simulink model "Linear_ADMIRE_sim"  (Simulink 8.4)
settings: Solver=ode4  StartTime=0.0  StopTime=10  FixedStep=dt  RelTol=1e-3
InitFcn:
  | INIT_LINEAR
values from neighbouring files (symbols this model uses):
  a1 = (180*d2r)/(80^3)    (= 6.13592315154e-06)    [INIT_LINEAR.m]    (also in INIT_NDI.m)
  a2 = (24*d2r)/(80^3)    (= 8.18123086872e-07)    [INIT_LINEAR.m]    (also in INIT_NDI.m)
  a3 = (5*d2r)/(200)    (= 0.000436332312999)    [INIT_LINEAR.m]    (also in INIT_NDI.m)
  Abare = [-0.0369710265542 -0.00338320638614 0 0 0.00101076287488 0 0 0 0 1.00000000002 0 1.7763568394e-12 ... (784 elements, 28x28)]    [Trim_M0p22ALT20_LinDATA.mat]    (also in Trim_M0p3ALT2000_LinDATA.mat = [-0.0208061645292 -0.00191640084378 0 0 0.000610808752105 0 )
  Bbare = [-1.10043807057 0.00182125944543 -0.00701366565749 0.707306131876 1.12037014439 -0.330899025785 0 0 0 0 0 0 ... (448 elements, 28x16)]    [Trim_M0p22ALT20_LinDATA.mat]    (also in Trim_M0p3ALT2000_LinDATA.mat = [-1.42042676365 -0.000549876720984 -0.00633411409606 0.84954)
  CAmethod = 1    [ACA_init.m]    (also in INIT_LINEAR.m = 0; INIT_NDI.m = 0)
  Canard_max = interp1(M_vec,[25 25 25 15 15 15 15 15]*d2r,Mach,'next')    [INIT_LINEAR.m]    (also in INIT_NDI.m = [25 25 25 15 15 15 15 15]*d2r)
  Canard_min = interp1(M_vec,[-55 -55 -25 -15 -15 -15 -15 -15]*d2r,Mach,'next')    [INIT_LINEAR.m]    (also in INIT_NDI.m = [-55 -55 -25 -15 -15 -15 -15 -15]*d2r)
  CAobm = CAobm(:,1:12)    [INIT_LINEAR.m]
  Cbare = [1 0 0 0 0 0 0 0 0 0 0 0 ... (1652 elements, 59x28)]    [Trim_M0p22ALT20_LinDATA.mat]    (also in Trim_M0p3ALT2000_LinDATA.mat)
  CBobm = CCV*Bbare    [INIT_LINEAR.m]
  Dbare = [0 0 0 0 0 0 0 0 0 0 0 0 ... (944 elements, 59x16)]    [Trim_M0p22ALT20_LinDATA.mat]    (also in Trim_M0p3ALT2000_LinDATA.mat)
  dt = 0.01    [ACA_init.m]    (also in INIT_LINEAR.m; INIT_NDI.m)
  DTY_max = 0.002    [ACA_init.m]    (also in INIT_LINEAR.m; INIT_NDI.m)
  DTY_min = -0.002    [ACA_init.m]    (also in INIT_LINEAR.m; INIT_NDI.m)
  DTZ_max = 0.002    [ACA_init.m]    (also in INIT_LINEAR.m; INIT_NDI.m)
  DTZ_min = -0.002    [ACA_init.m]    (also in INIT_LINEAR.m; INIT_NDI.m)
  Elevon_max = interp1(M_vec,[30 30 25 25 25 25 25 25]*d2r,Mach,'next')    [INIT_LINEAR.m]    (also in INIT_NDI.m = [30 30 25 25 25 25 25 25]*d2r)
  Elevon_min = interp1(M_vec,[-30 -30 -30 -30 -30 -30 -30 -30]*d2r,Mach,'next')    [INIT_LINEAR.m]    (also in INIT_NDI.m = [-30 -30 -30 -30 -30 -30 -30 -30]*d2r)
  Fas_t = [0 1 1+dt 2. 2.+dt 8]    [INIT_LINEAR.m]
  Fas_v = [0 0 1 1 0 0]*40*0    [INIT_LINEAR.m]
  Fes_t = [0 1 1+dt 4 4+dt 7 7+dt 8]    [INIT_LINEAR.m]
  Fes_v = [0 0 1 1 -1 -1 0 0]*40    [INIT_LINEAR.m]
  Frp_t = [0 1 1+dt 6. 6.+dt 8]    [INIT_LINEAR.m]
  Frp_v = [0 0 1 1 0 0]*100*0    [INIT_LINEAR.m]
  G = [ 0 1 0 ... (first row only)    [ACA_init.m]    (also in INIT_LINEAR.m = [ 1 0 0; INIT_NDI.m)
  Kfb = -1.71    [INIT_LINEAR.m]
  Kfq = -3.4    [INIT_LINEAR.m]
  Kib = 5.14    [INIT_LINEAR.m]
  Kiq = 4    [INIT_LINEAR.m]
  Kp = 2.    (= 2)    [INIT_LINEAR.m]
  Kpb = 4.29    [INIT_LINEAR.m]
  Kpq = 3.4    [INIT_LINEAR.m]
  Kr = 14    [INIT_LINEAR.m]
  LEF_max = interp1(M_vec,[30 30 30 20 20 15 10 10]*d2r,Mach,'next')    [INIT_LINEAR.m]    (also in INIT_NDI.m = [30 30 30 20 20 15 10 10]*d2r)
  LEF_min = interp1(M_vec,[-10 -10 -10 -10 -10 -10 -10 -10]*d2r,Mach,'next')    [INIT_LINEAR.m]    (also in INIT_NDI.m = [-10 -10 -10 -10 -10 -10 -10 -10]*d2r)
  LG_max = 1    [ACA_init.m]    (also in INIT_LINEAR.m; INIT_NDI.m)
  LG_min = 0    [ACA_init.m]    (also in INIT_LINEAR.m; INIT_NDI.m)
  LPmethod = 3    [ACA_init.m]    (also in INIT_LINEAR.m = 0; INIT_NDI.m = 0; LPwrap.m = 0; LPwrap_1.m = 0)
  NumU = 16    [ACA_init.m]    (also in INIT_LINEAR.m; INIT_NDI.m; test.m; test_LPwrap.m)
  PD_max = 10    [ACA_init.m]    (also in INIT_LINEAR.m; INIT_NDI.m)
  PD_min = -10    [ACA_init.m]    (also in INIT_LINEAR.m; INIT_NDI.m)
  r2d = 180/pi    (= 57.2957795131)    [ACA_init.m]    (also in INIT_LINEAR.m; INIT_NDI.m)
  Rudder_max = interp1(M_vec,[30 30 25 20 15 15 15 10]*d2r,Mach,'next')    [INIT_LINEAR.m]    (also in INIT_NDI.m = [30 30 25 20 15 15 15 10]*d2r)
  Rudder_min = interp1(M_vec,[-30 -30 -25 -20 -15 -15 -15 -10]*d2r,Mach,'next')    [INIT_LINEAR.m]    (also in INIT_NDI.m = [-30 -30 -25 -20 -15 -15 -15 -10]*d2r)
  TSS_max = 1    [ACA_init.m]    (also in INIT_LINEAR.m; INIT_NDI.m)
  TSS_min = 0    [ACA_init.m]    (also in INIT_LINEAR.m; INIT_NDI.m)
  TSS_t = [0 1 1+dt 6. 6.+dt 8]    [INIT_LINEAR.m]
  TSS_v = [0 0 .1 .1 0 0]*0+u0new(10)    [INIT_LINEAR.m]
  UACTIVE = [ ... (first row only)    [INIT_LINEAR.m]
  UD_max = 10    [ACA_init.m]    (also in INIT_LINEAR.m; INIT_NDI.m)
  UD_min = -10    [ACA_init.m]    (also in INIT_LINEAR.m; INIT_NDI.m)
  Umax = [Canard_max*[1 1] Elevon_max*[1 1 1 1] Rudder_max LEF_max     LG_max TSS_max DTY_max DTZ_max UD_max VD_max WD_max PD_max]'    [INIT_LINEAR.m]    (also in INIT_NDI.m = [25 25 30 30 30 30 30]'*d2r)
  Umin = [Canard_min*[1 1] Elevon_min*[1 1 1 1] Rudder_min LEF_min     LG_min TSS_min DTY_min DTZ_min UD_min VD_min WD_min PD_min]'    [INIT_LINEAR.m]    (also in INIT_NDI.m = [-55 -55 -30 -30 -30 -30 -30]'*d2r)
  Unom = u0new    [INIT_LINEAR.m]
  Upref = [0 0 0 0 0 0 0 0 0 0 0 0 0 0 0 0]'    [ACA_init.m]    (also in INIT_LINEAR.m; INIT_NDI.m)
  UsePref = 0    [INIT_LINEAR.m]
  VD_max = 10    [ACA_init.m]    (also in INIT_LINEAR.m; INIT_NDI.m)
  VD_min = -10    [ACA_init.m]    (also in INIT_LINEAR.m; INIT_NDI.m)
  WD_max = 10    [ACA_init.m]    (also in INIT_LINEAR.m; INIT_NDI.m)
  WD_min = -10    [ACA_init.m]    (also in INIT_LINEAR.m; INIT_NDI.m)
  Wp = W'*W    [ACA_init.m]    (also in INIT_LINEAR.m; INIT_NDI.m; test.m; test_LPwrap.m)
  y0bare = [74.8477877145 0.159877852888 0 0 0 0 0 0.159877852888 0 0 0 -20 ... (73 elements, 73x1)]    [Trim_M0p22ALT20_LinDATA.mat]    (also in Trim_M0p3ALT2000_LinDATA.mat = [99.7587452043 0.116024082006 0 0 0 0 0 0.116024082006 0 0 0)
undefined symbols (not defined in the file or in its folder): CGIwrap, DAwrap, LPwrap, VJAwrap
libraries: simulink x6
(part 1 of 2)
settings Model: Creator=kenbordignon  LastModifiedBy=bordignk
settings DebuggingCC: CheckSSInitialOutputMsg=off  SolverPrmCheckMsg=none  UnconnectedInputMsg=none  UnconnectedOutputMsg=none  UnconnectedLineMsg=none

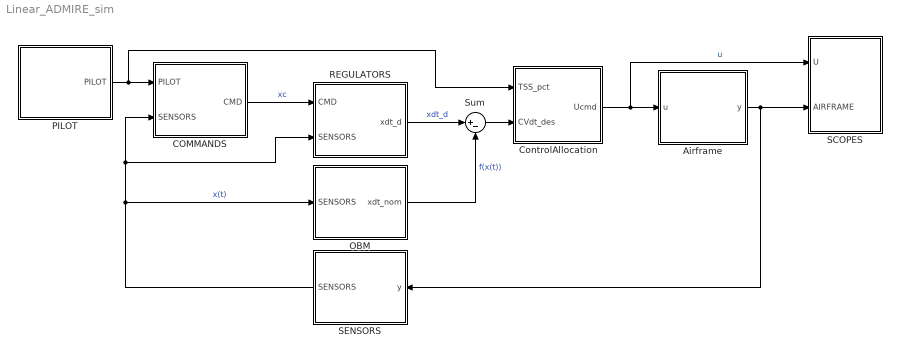
== system Linear_ADMIRE_sim ==
  Airframe : Subsystem
      mask Display: disp('AIRFRAME')
  COMMANDS : Subsystem
      mask Display: disp('COMMANDS')
  ControlAllocation : Subsystem
      mask Display: disp('CONTOL\nALLOCATION')
  OBM : Subsystem
      mask Display: disp('ON-BOARD\nMODEL')
  PILOT : Subsystem
      mask Display: disp('PILOT\nINCEPTORS')
  REGULATORS : Subsystem
      mask Display: disp('REGULATORS')
  SCOPES : Subsystem
      mask Display: disp('SCOPES\n&\nDISPLAYS')
  SENSORS : Subsystem
      mask Display: disp('SENSORS')
  Sum : Sum  Inputs=|+-
  wires:
  Airframe/1(y) -> SENSORS/1(y), SCOPES/2(AIRFRAME)
  SENSORS/1(SENSORS) -> OBM/1(SENSORS), REGULATORS/2(SENSORS), COMMANDS/2(SENSORS)  "x(t)"
  REGULATORS/1(xdt_d) -> Sum/1  "xdt_d"
  Sum/1 -> ControlAllocation/2(CVdt_des)
  COMMANDS/1(CMD) -> REGULATORS/1(CMD)  "xc"
  PILOT/1(PILOT) -> ControlAllocation/1(TSS_pct), COMMANDS/1(PILOT)
  ControlAllocation/1(Ucmd) -> Airframe/1(u), SCOPES/1(U)  "u"
  OBM/1(xdt_nom) -> Sum/2  "f(x(t))"

== system Linear_ADMIRE_sim/Airframe ==
  u : Inport
  A : Subsystem
      mask Display: disp('A')
  B : Subsystem
      mask Display: disp('B')
  C : Subsystem
      mask Display: disp('C')
  Constant4 : Constant  Value=Unom
  D : Subsystem
      mask Display: disp('D')
  Integrator : Integrator
  Sum : Sum  Inputs=|++
  Sum1 : Sum  Inputs=++|
  Sum2 : Sum  Inputs=|+-
  y : Outport
  wires:
  Integrator/1 -> C/1(In1), A/1(In1)  "x"
  B/1(Out1) -> Sum/1
  Sum/1 -> Integrator/1  "xdt"
  A/1(Out1) -> Sum/2
  Sum2/1 -> B/1(In1), D/1(In1)  "u"
  D/1(Out1) -> Sum1/1
  C/1(Out1) -> Sum1/2
  Sum1/1 -> y/1  "y"
  u/1 -> Sum2/1  "u"
  Constant4/1 -> Sum2/2

== system Linear_ADMIRE_sim/COMMANDS ==
  PILOT : Inport
  SENSORS : Inport  Port=2
  Bus Creator : BusCreator  Inputs=3
  PitchCmd : Subsystem
  RollCmd : Subsystem
  YawCmd : Subsystem
  CMD : Outport
  wires:
  PILOT/1 -> RollCmd/1(PILOT), YawCmd/1(PILOT), PitchCmd/1(PILOT)
  Bus Creator/1 -> CMD/1
  PitchCmd/1(Qc) -> Bus Creator/2
  RollCmd/1(Pc) -> Bus Creator/1
  YawCmd/1(Rc) -> Bus Creator/3
  SENSORS/1 -> YawCmd/2(SENSORS)

== system Linear_ADMIRE_sim/ControlAllocation ==
  TSS_pct : Inport
  CVdt_des : Inport  Port=2
  Bus Selector : BusSelector  OutputSignals=TSS_pct
  GetU : Subsystem
  PostProcess : Subsystem
  PreProcess : Subsystem
  Ucmd : Outport
  wires:
  PreProcess/1(PrePro) -> GetU/1(PrePro), PostProcess/2(PrePro)
  GetU/1(u) -> PostProcess/1(u)
  CVdt_des/1 -> PreProcess/1(CVdt_des)  "CVdt_des"
  PostProcess/1(Ucmd) -> Ucmd/1
  TSS_pct/1 -> Bus Selector/1
  Bus Selector/1 -> PostProcess/3(TSS_pct)  "<TSS_pct>"

== system Linear_ADMIRE_sim/OBM ==
  SENSORS : Inport
  Bus Selector : BusSelector  OutputSignals=VT_mps,ALPHA_rad,BETA_rad,P_rps,Q_rps,R_rps,PSI_rad,THETA_rad,PHI_rad,X_m,Y_m,Z_m  OutputAsBus=on
  Bus to Vector : BusToVector
  Gain1 : Gain  Gain=CAobm  Multiplication=Matrix(K*u)
  xdt_nom : Outport
  wires:
  SENSORS/1 -> Bus Selector/1
  Gain1/1 -> xdt_nom/1  "xdt_nom"
  Bus Selector/1 -> Bus to Vector/1  "x"
  Bus to Vector/1 -> Gain1/1

== system Linear_ADMIRE_sim/PILOT ==
  1-D Lookup Table : Lookup_n-D  NumberOfTableDimensions=1  BreakpointsForDimension1=Fas_t  Table=Fas_v  ExtrapMethod=Clip  UseLastTableValue=on  RndMeth=Simplest  InputSameDT=on
  1-D Lookup Table1 : Lookup_n-D  NumberOfTableDimensions=1  BreakpointsForDimension1=Fes_t  Table=Fes_v  ExtrapMethod=Clip  UseLastTableValue=on  RndMeth=Simplest  InputSameDT=on
  1-D Lookup Table2 : Lookup_n-D  NumberOfTableDimensions=1  BreakpointsForDimension1=Frp_t  Table=Frp_v  ExtrapMethod=Clip  UseLastTableValue=on  RndMeth=Simplest  InputSameDT=on
  1-D Lookup Table3 : Lookup_n-D  NumberOfTableDimensions=1  BreakpointsForDimension1=TSS_t  Table=TSS_v  ExtrapMethod=Clip  UseLastTableValue=on  RndMeth=Simplest  InputSameDT=on
  Bus Creator : BusCreator
  Clock : Clock
  Saturation : Saturate  UpperLimit=80  LowerLimit=-80
  Saturation1 : Saturate  UpperLimit=80  LowerLimit=-40
  Saturation2 : Saturate  UpperLimit=200  LowerLimit=-200
  Saturation3 : Saturate  UpperLimit=1  LowerLimit=0
  PILOT : Outport
  wires:
  Clock/1 -> 1-D Lookup Table/1, 1-D Lookup Table1/1, 1-D Lookup Table2/1, 1-D Lookup Table3/1
  1-D Lookup Table1/1 -> Saturation1/1
  1-D Lookup Table2/1 -> Saturation2/1
  1-D Lookup Table3/1 -> Saturation3/1
  Bus Creator/1 -> PILOT/1  "PILOT"
  Saturation/1 -> Bus Creator/1  "Fas_N"
  Saturation1/1 -> Bus Creator/2  "Fes_N"
  Saturation2/1 -> Bus Creator/3  "Frp_N"
  Saturation3/1 -> Bus Creator/4  "TSS_pct"
  1-D Lookup Table/1 -> Saturation/1

== system Linear_ADMIRE_sim/REGULATORS ==
  CMD : Inport
  SENSORS : Inport  Port=2
  Mux : Mux  Inputs=3
  PitchReg : Subsystem
  RollReg : Subsystem
  YawReg : Subsystem
  xdt_d : Outport
  wires:
  RollReg/1(Pdt_d) -> Mux/1
  PitchReg/1(Qdt_d) -> Mux/2
  YawReg/1(Rdt_d) -> Mux/3
  CMD/1 -> RollReg/1(CMD), PitchReg/1(CMD), YawReg/1(CMD)
  Mux/1 -> xdt_d/1  "xdt_d"
  SENSORS/1 -> RollReg/2(SENSORS), PitchReg/2(SENSORS), YawReg/2(SENSORS)

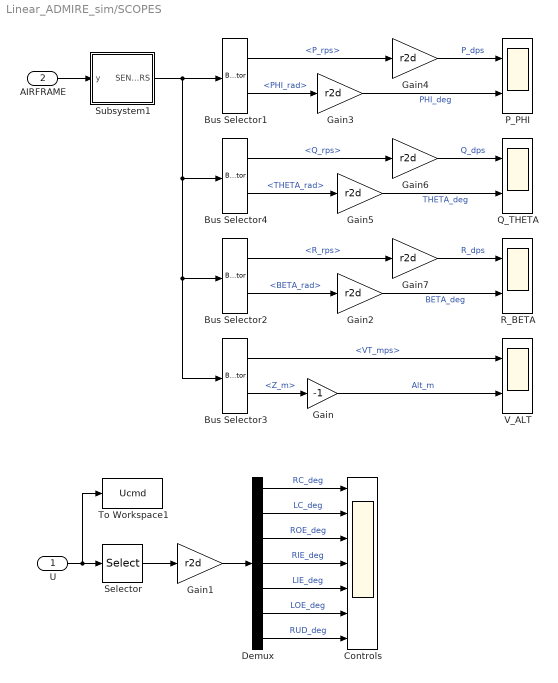
== system Linear_ADMIRE_sim/SCOPES ==
  U : Inport
  AIRFRAME : Inport  Port=2
  Bus Selector1 : BusSelector  OutputSignals=P_rps,PHI_rad
  Bus Selector2 : BusSelector  OutputSignals=R_rps,BETA_rad
  Bus Selector3 : BusSelector  OutputSignals=VT_mps,Z_m
  Bus Selector4 : BusSelector  OutputSignals=Q_rps,THETA_rad
  Controls : Scope  NumInputPorts=7
      settings: TimeRange=10  YMin=-10~-10~-5~-5~-5~-5~-5  YMax=5~5~5~5~5~5~5  SaveName=ScopeData2
  Demux : Demux  Outputs=7
  Gain : Gain  Gain=-1
  Gain{1..7} (7 alike) : Gain  Gain=r2d
  P_PHI : Scope  NumInputPorts=2
      settings: TimeRange=10  YMin=0~0  YMax=20~30
  Q_THETA : Scope  NumInputPorts=2
      settings: TimeRange=10  YMin=-4~8  YMax=4~18  SaveName=ScopeData4
  R_BETA : Scope  NumInputPorts=2
      settings: TimeRange=10  YMin=-10~-1  YMax=10~3
  Selector : Selector  InputPortWidth=16  Indices=[1:7]
  Subsystem1 : Subsystem
  To Workspace1 : ToWorkspace  VariableName=Ucmd  SampleTime=-1
  V_ALT : Scope  NumInputPorts=2
      settings: TimeRange=10  YMin=70~10  YMax=76~50  SaveName=ScopeData3
  wires:
  Subsystem1/1(SENSORS) -> Bus Selector3/1, Bus Selector2/1, Bus Selector4/1, Bus Selector1/1
  Bus Selector1/1 -> Gain4/1  "<P_rps>"
  AIRFRAME/1 -> Subsystem1/1(y)
  Bus Selector2/2 -> Gain2/1  "<BETA_rad>"
  Bus Selector1/2 -> Gain3/1  "<PHI_rad>"
  Bus Selector3/1 -> V_ALT/1  "<VT_mps>"
  Bus Selector3/2 -> Gain/1  "<Z_m>"
  Gain/1 -> V_ALT/2  "Alt_m"
  Selector/1 -> Gain1/1
  U/1 -> Selector/1, To Workspace1/1
  Demux/2 -> Controls/2  "LC_deg"
  Demux/3 -> Controls/3  "ROE_deg"
  Demux/4 -> Controls/4  "RIE_deg"
  Demux/5 -> Controls/5  "LIE_deg"
  Demux/6 -> Controls/6  "LOE_deg"
  Demux/7 -> Controls/7  "RUD_deg"
  Gain1/1 -> Demux/1
  Gain2/1 -> R_BETA/2  "BETA_deg"
  Gain3/1 -> P_PHI/2  "PHI_deg"
  Gain4/1 -> P_PHI/1  "P_dps"
  Bus Selector4/1 -> Gain6/1  "<Q_rps>"
  Bus Selector4/2 -> Gain5/1  "<THETA_rad>"
  Gain5/1 -> Q_THETA/2  "THETA_deg"
  Gain6/1 -> Q_THETA/1  "Q_dps"
  Gain7/1 -> R_BETA/1  "R_dps"
  Bus Selector2/1 -> Gain7/1  "<R_rps>"
  Demux/1 -> Controls/1  "RC_deg"

== system Linear_ADMIRE_sim/SENSORS ==
  note: Select 1:12 for actual values
      |
      | Select 32:43 for sensor approximations
  y : Inport
  Bus Creator : BusCreator  Inputs=12
  Demux : Demux  Outputs=12
  Selector : Selector  InputPortWidth=59  Indices=SensorIDX
  Unit Delay : UnitDelay  SampleTime=dt
  SENSORS : Outport
  wires:
  Demux/1 -> Bus Creator/1  "VT_mps"
  Demux/2 -> Bus Creator/2  "ALPHA_rad"
  Demux/3 -> Bus Creator/3  "BETA_rad"
  Demux/4 -> Bus Creator/4  "P_rps"
  Demux/5 -> Bus Creator/5  "Q_rps"
  Demux/6 -> Bus Creator/6  "R_rps"
  Demux/7 -> Bus Creator/7  "PSI_rad"
  Demux/8 -> Bus Creator/8  "THETA_rad"
  Demux/9 -> Bus Creator/9  "PHI_rad"
  Demux/10 -> Bus Creator/10  "X_m"
  Demux/11 -> Bus Creator/11  "Y_m"
  Demux/12 -> Bus Creator/12  "Z_m"
  y/1 -> Unit Delay/1
  Bus Creator/1 -> SENSORS/1
  Selector/1 -> Demux/1
  Unit Delay/1 -> Selector/1

== system Linear_ADMIRE_sim/Airframe/A ==
  In1 : Inport
  Gain1 : Gain  Gain=Abare  Multiplication=Matrix(K*u)
  Out1 : Outport
  wires:
  In1/1 -> Gain1/1
  Gain1/1 -> Out1/1

== system Linear_ADMIRE_sim/Airframe/B ==
  In1 : Inport
  Gain : Gain  Gain=Bbare  Multiplication=Matrix(K*u)
  Out1 : Outport
  wires:
  In1/1 -> Gain/1
  Gain/1 -> Out1/1

== system Linear_ADMIRE_sim/Airframe/C ==
  In1 : Inport
  Gain3 : Gain  Gain=Cbare  Multiplication=Matrix(K*u)
  Out1 : Outport
  wires:
  In1/1 -> Gain3/1
  Gain3/1 -> Out1/1

== system Linear_ADMIRE_sim/Airframe/D ==
  In1 : Inport
  Gain2 : Gain  Gain=Dbare  Multiplication=Matrix(K*u)
  Out1 : Outport
  wires:
  In1/1 -> Gain2/1
  Gain2/1 -> Out1/1

== system Linear_ADMIRE_sim/COMMANDS/PitchCmd ==
  PILOT : Inport
  Bus Selector1 : BusSelector  OutputSignals=Fes_N
  QCMD_Gradient : Lookup_n-D  NumberOfTableDimensions=1  BreakpointsForDimension1=[-80:80]  Table=a2*([-80:80].^3)  ExtrapMethod=Clip  UseLastTableValue=on  RndMeth=Simplest  InputSameDT=on
  Qc : Outport
  wires:
  PILOT/1 -> Bus Selector1/1
  Bus Selector1/1 -> QCMD_Gradient/1  "<Fes_N>"
  QCMD_Gradient/1 -> Qc/1  "Qc_rps"

== system Linear_ADMIRE_sim/COMMANDS/RollCmd ==
  PILOT : Inport
  Bus Selector2 : BusSelector  OutputSignals=Fas_N
  Gain4 : Gain  Gain=r2d
  PCMD_Gradient : Lookup_n-D  NumberOfTableDimensions=1  BreakpointsForDimension1=[-80:80]  Table=a1*([-80:80].^3)  ExtrapMethod=Clip  UseLastTableValue=on  RndMeth=Simplest  InputSameDT=on
  PC_dps : Scope
      settings: TimeRange=10  YMin=-50  YMax=50  SaveName=ScopeData8
  Pc : Outport
  wires:
  PILOT/1 -> Bus Selector2/1
  Bus Selector2/1 -> PCMD_Gradient/1  "<Fas_N>"
  PCMD_Gradient/1 -> Pc/1, Gain4/1  "Pc_rps"
  Gain4/1 -> PC_dps/1

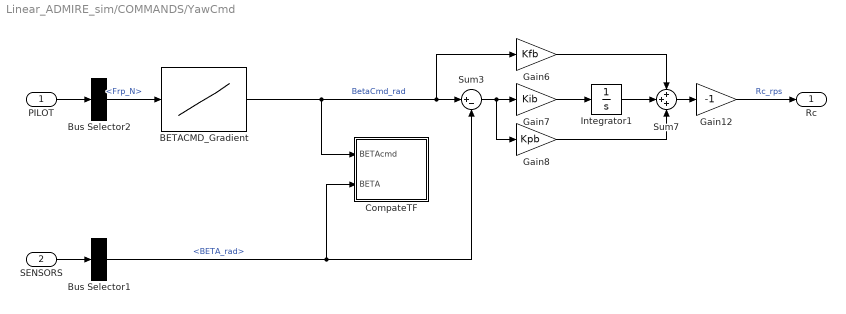
== system Linear_ADMIRE_sim/COMMANDS/YawCmd ==
  PILOT : Inport
  SENSORS : Inport  Port=2
  BETACMD_Gradient : Lookup_n-D  NumberOfTableDimensions=1  BreakpointsForDimension1=[-200 200]  Table=a3*([-200 200])  ExtrapMethod=Clip  UseLastTableValue=on  RndMeth=Simplest  InputSameDT=on
  Bus Selector1 : BusSelector  OutputSignals=BETA_rad
  Bus Selector2 : BusSelector  OutputSignals=Frp_N
  CompateTF : Subsystem
  Gain12 : Gain  Gain=-1
  Gain6 : Gain  Gain=Kfb
  Gain7 : Gain  Gain=Kib
  Gain8 : Gain  Gain=Kpb
  Integrator1 : Integrator
  Sum3 : Sum  Inputs=|+-
  Sum7 : Sum  Inputs=+++
  Rc : Outport
  wires:
  Sum7/1 -> Gain12/1
  Gain6/1 -> Sum7/1
  Gain7/1 -> Integrator1/1
  Sum3/1 -> Gain7/1, Gain8/1
  Gain8/1 -> Sum7/3
  Integrator1/1 -> Sum7/2
  Gain12/1 -> Rc/1  "Rc_rps"
  PILOT/1 -> Bus Selector2/1
  SENSORS/1 -> Bus Selector1/1
  Bus Selector1/1 -> Sum3/2, CompateTF/2(BETA)  "<BETA_rad>"
  Bus Selector2/1 -> BETACMD_Gradient/1  "<Frp_N>"
  BETACMD_Gradient/1 -> Sum3/1, Gain6/1, CompateTF/1(BETAcmd)  "BetaCmd_rad"

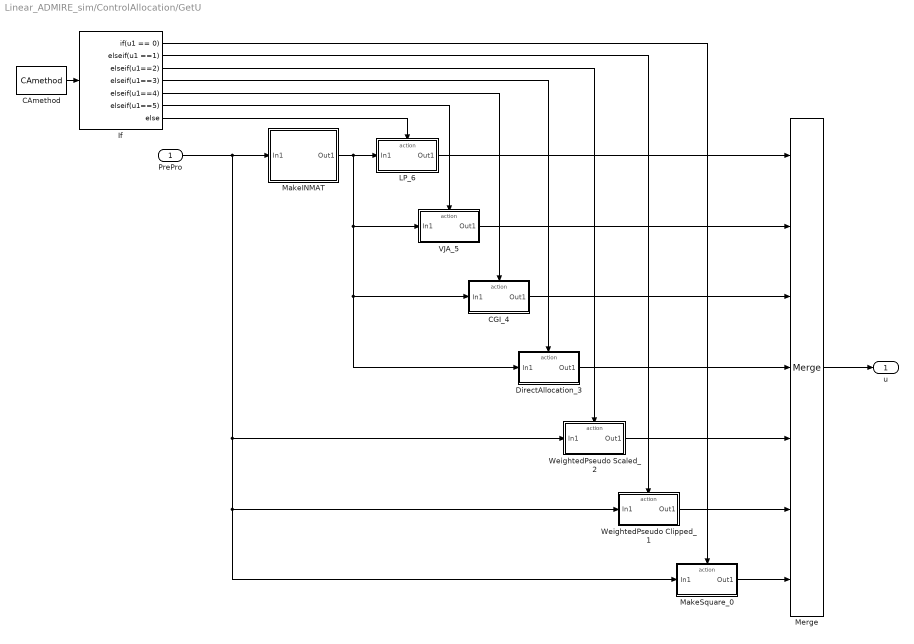
== system Linear_ADMIRE_sim/ControlAllocation/GetU ==
  PrePro : Inport
  CAmethod : Constant  Value=CAmethod  OutDataTypeStr=int8
  CGI_4 : Subsystem  TreatAsAtomicUnit=on
  DirectAllocation_3 : Subsystem  TreatAsAtomicUnit=on
  If : If  IfExpression=u1 == 0  ElseIfExpressions=u1 ==1, u1==2, u1==3, u1==4, u1==5
  LP_6 : Subsystem  TreatAsAtomicUnit=on
  MakeINMAT : Subsystem
  MakeSquare_0 : Subsystem  TreatAsAtomicUnit=on
  Merge : Merge  Inputs=7
  VJA_5 : Subsystem  TreatAsAtomicUnit=on
  WeightedPseudo Clipped_1 : Subsystem  TreatAsAtomicUnit=on
  WeightedPseudo Scaled_2 : Subsystem  TreatAsAtomicUnit=on
  u : Outport
  wires:
  CAmethod/1 -> If/1
  If/1 -> MakeSquare_0/Action
  If/2 -> WeightedPseudo Clipped_1/Action
  If/3 -> WeightedPseudo Scaled_2/Action
  If/4 -> DirectAllocation_3/Action
  VJA_5/1(Out1) -> Merge/2
  MakeSquare_0/1(Out1) -> Merge/7
  WeightedPseudo Clipped_1/1(Out1) -> Merge/6
  WeightedPseudo Scaled_2/1(Out1) -> Merge/5
  DirectAllocation_3/1(Out1) -> Merge/4
  If/5 -> CGI_4/Action
  CGI_4/1(Out1) -> Merge/3
  If/6 -> VJA_5/Action
  Merge/1 -> u/1
  If/7 -> LP_6/Action
  LP_6/1(Out1) -> Merge/1
  PrePro/1 -> MakeINMAT/1(In1), WeightedPseudo Scaled_2/1(In1), WeightedPseudo Clipped_1/1(In1), MakeSquare_0/1(In1)
  MakeINMAT/1(Out1) -> LP_6/1(In1), VJA_5/1(In1), DirectAllocation_3/1(In1), CGI_4/1(In1)

== system Linear_ADMIRE_sim/ControlAllocation/PostProcess ==
  u : Inport
  PrePro : Inport  Port=2
  TSS_pct : Inport  Port=3
  Bus Selector1 : BusSelector  OutputSignals=Unom
  DriveToPreferred : Subsystem
  LimitCommands : Subsystem
  Sum2 : Sum  Inputs=|++
  Sum3 : Sum  Inputs=|++
  Ucmd : Outport
  wires:
  Sum2/1 -> Sum3/1
  Sum3/1 -> LimitCommands/1(In1)
  u/1 -> DriveToPreferred/2(u), Sum2/1
  PrePro/1 -> DriveToPreferred/1(PrePro), Bus Selector1/1
  LimitCommands/1(Ucmd) -> Ucmd/1
  Bus Selector1/1 -> Sum2/2  "<Unom>"
  DriveToPreferred/1(Out2) -> Sum3/2
  TSS_pct/1 -> LimitCommands/2(TSS_pct)

== system Linear_ADMIRE_sim/ControlAllocation/PreProcess ==
  note: Data which usually comes from an
      | On-board Model and is assumed
      | constant for this simulation
  CVdt_des : Inport
  Bus Creator : BusCreator  Inputs=6
  Bus Creator1 : BusCreator
  Bus Selector1 : BusSelector  OutputSignals=CB,Unom,Umax,Umin
  Constant : Constant  Value=UACTIVE
  Constant1 : Constant  Value=CBobm
  Constant2 : Constant  Value=Umax
  Constant3 : Constant  Value=Umin
  Constant4 : Constant  Value=Unom
  PrePro : Outport
  wires:
  CVdt_des/1 -> Bus Creator/1
  Bus Creator/1 -> PrePro/1
  Constant/1 -> Bus Creator/6  "INDX"
  Constant1/1 -> Bus Creator1/1  "CB"
  Constant2/1 -> Bus Creator1/2  "Umax"
  Constant3/1 -> Bus Creator1/3  "Umin"
  Constant4/1 -> Bus Creator1/4  "Unom"
  Bus Creator1/1 -> Bus Selector1/1
  Bus Selector1/1 -> Bus Creator/2  "<CB>"
  Bus Selector1/2 -> Bus Creator/3  "<Unom>"
  Bus Selector1/3 -> Bus Creator/4  "<Umax>"
  Bus Selector1/4 -> Bus Creator/5  "<Umin>"

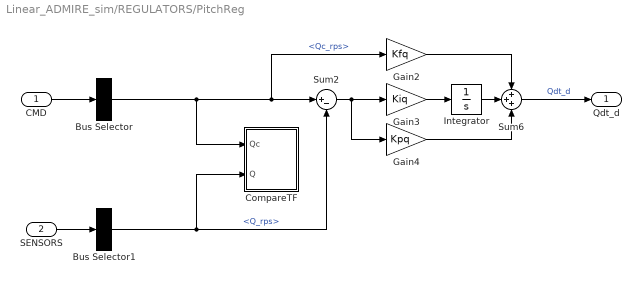
== system Linear_ADMIRE_sim/REGULATORS/PitchReg ==
  CMD : Inport
  SENSORS : Inport  Port=2
  Bus Selector : BusSelector  OutputSignals=Qc_rps
  Bus Selector1 : BusSelector  OutputSignals=Q_rps
  CompareTF : Subsystem
  Gain2 : Gain  Gain=Kfq
  Gain3 : Gain  Gain=Kiq
  Gain4 : Gain  Gain=Kpq
  Integrator : Integrator
  Sum2 : Sum  Inputs=|+-
  Sum6 : Sum  Inputs=+++
  Qdt_d : Outport
  wires:
  Sum2/1 -> Gain3/1, Gain4/1
  Gain3/1 -> Integrator/1
  Integrator/1 -> Sum6/2
  Gain4/1 -> Sum6/3
  Gain2/1 -> Sum6/1
  Bus Selector1/1 -> Sum2/2, CompareTF/2(Q)  "<Q_rps>"
  SENSORS/1 -> Bus Selector1/1
  Bus Selector/1 -> Sum2/1, Gain2/1, CompareTF/1(Qc)  "<Qc_rps>"
  Sum6/1 -> Qdt_d/1  "Qdt_d"
  CMD/1 -> Bus Selector/1

== system Linear_ADMIRE_sim/REGULATORS/RollReg ==
  CMD : Inport
  SENSORS : Inport  Port=2
  Bus Selector : BusSelector  OutputSignals=Pc_rps
  Bus Selector1 : BusSelector  OutputSignals=P_rps
  CompareTF : Subsystem
  Gain : Gain  Gain=Kp
  Sum8 : Sum  Inputs=|+-
  Pdt_d : Outport
  wires:
  Sum8/1 -> Gain/1
  Bus Selector1/1 -> Sum8/2, CompareTF/2(P)  "<P_rps>"
  SENSORS/1 -> Bus Selector1/1
  Gain/1 -> Pdt_d/1  "Pdt_d"
  CMD/1 -> Bus Selector/1
  Bus Selector/1 -> Sum8/1, CompareTF/1(Pc)  "<Pc_rps>"

== system Linear_ADMIRE_sim/REGULATORS/YawReg ==
  CMD : Inport
  SENSORS : Inport  Port=2
  Bus Selector : BusSelector  OutputSignals=Rc_rps
  Bus Selector1 : BusSelector  OutputSignals=R_rps
  CompareTF : Subsystem
  Gain5 : Gain  Gain=Kr
  Sum4 : Sum  Inputs=|+-
  Rdt_d : Outport
  wires:
  Sum4/1 -> Gain5/1
  Gain5/1 -> Rdt_d/1  "Rdt_d"
  CMD/1 -> Bus Selector/1
  SENSORS/1 -> Bus Selector1/1
  Bus Selector1/1 -> CompareTF/2(R), Sum4/2  "<R_rps>"
  Bus Selector/1 -> Sum4/1, CompareTF/1(Rc)  "<Rc_rps>"

== system Linear_ADMIRE_sim/SCOPES/Subsystem1 ==
  note: Select 1:12 for actual values
      |
      | Select 32:43 for sensor approximations
  note: Add in the trim conditions
  y : Inport
  Bus Creator : BusCreator  Inputs=12
  Constant : Constant  Value=y0bare(1:12)
  Demux : Demux  Outputs=12
  Selector : Selector  InputPortWidth=59  Indices=[1:12]
  Sum : Sum  Inputs=|++
  SENSORS : Outport
  wires:
  Demux/1 -> Bus Creator/1  "VT_mps"
  Demux/2 -> Bus Creator/2  "ALPHA_rad"
  Demux/3 -> Bus Creator/3  "BETA_rad"
  Demux/4 -> Bus Creator/4  "P_rps"
  Demux/5 -> Bus Creator/5  "Q_rps"
  Demux/6 -> Bus Creator/6  "R_rps"
  Demux/7 -> Bus Creator/7  "PSI_rad"
  Demux/8 -> Bus Creator/8  "THETA_rad"
  Demux/9 -> Bus Creator/9  "PHI_rad"
  Demux/10 -> Bus Creator/10  "X_m"
  Demux/11 -> Bus Creator/11  "Y_m"
  Demux/12 -> Bus Creator/12  "Z_m"
  y/1 -> Selector/1
  Bus Creator/1 -> SENSORS/1
  Sum/1 -> Demux/1
  Constant/1 -> Sum/2
  Selector/1 -> Sum/1

== system Linear_ADMIRE_sim/COMMANDS/YawCmd/CompateTF ==
  BETAcmd : Inport
  BETA : Inport  Port=2
  BetaTF_Beta : Scope
      settings: TimeRange=10  YMin=-1  YMax=3  SaveName=ScopeData6
  Gain2 : Gain  Gain=r2d
  Gain3 : Gain  Gain=r2d
  Mux1 : Mux  Inputs=2
  Scope2 : Scope
      settings: TimeRange=10  YMin=-6  YMax=1  SaveName=ScopeData7
  Sum2 : Sum  Inputs=|+-
  Transfer Fcn : TransferFcn  Numerator=[Kr*(Kfb+Kpb) Kr*Kib]  Denominator=[1 Kr Kr*Kpb Kr*Kib]
  Unit Delay : UnitDelay  SampleTime=dt
  wires:
  Mux1/1 -> Gain3/1
  Transfer Fcn/1 -> Unit Delay/1
  Sum2/1 -> Gain2/1
  Gain2/1 -> Scope2/1
  Gain3/1 -> BetaTF_Beta/1
  BETAcmd/1 -> Transfer Fcn/1
  BETA/1 -> Mux1/2, Sum2/2
  Unit Delay/1 -> Mux1/1, Sum2/1

== system Linear_ADMIRE_sim/ControlAllocation/GetU/CGI_4 ==
  In1 : Inport
  Action Port : ActionPort  ActionType=elseif
  MATLAB Fcn : MATLABFcn  MATLABFcn=CGIwrap(u)
  Out1 : Outport
  wires:
  MATLAB Fcn/1 -> Out1/1
  In1/1 -> MATLAB Fcn/1

== system Linear_ADMIRE_sim/ControlAllocation/GetU/DirectAllocation_3 ==
  In1 : Inport
  Action Port : ActionPort  ActionType=elseif
  MATLAB Fcn : MATLABFcn  MATLABFcn=DAwrap(u)
  Out1 : Outport
  wires:
  MATLAB Fcn/1 -> Out1/1
  In1/1 -> MATLAB Fcn/1

== system Linear_ADMIRE_sim/ControlAllocation/GetU/LP_6 ==
  In1 : Inport
  Action Port : ActionPort  ActionType=else
  MATLAB Fcn : MATLABFcn  MATLABFcn=LPwrap(u)
  Out1 : Outport
  wires:
  MATLAB Fcn/1 -> Out1/1
  In1/1 -> MATLAB Fcn/1

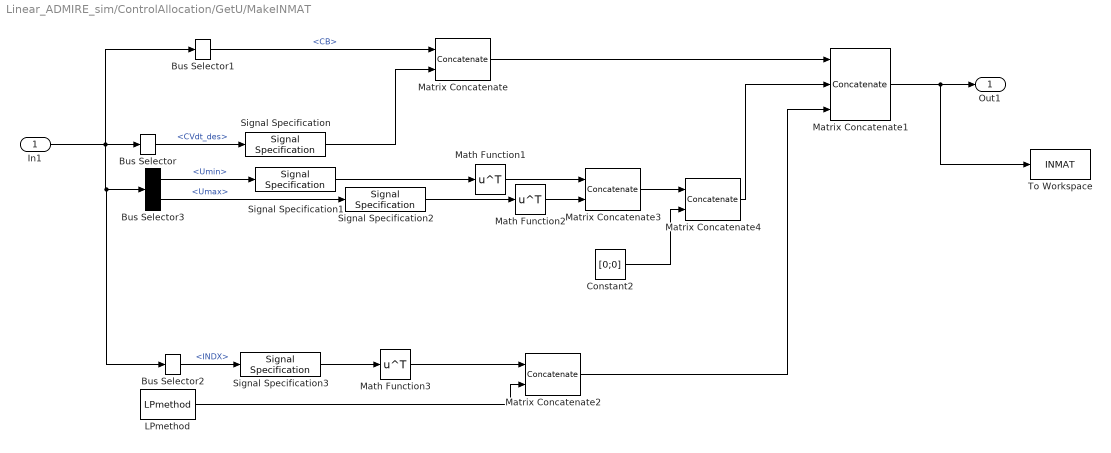
== system Linear_ADMIRE_sim/ControlAllocation/GetU/MakeINMAT ==
  In1 : Inport
  Bus Selector : BusSelector  OutputSignals=CVdt_des
  Bus Selector1 : BusSelector  OutputSignals=CB
  Bus Selector2 : BusSelector  OutputSignals=INDX
  Bus Selector3 : BusSelector  OutputSignals=Umin,Umax
  Constant2 : Constant  Value=[0;0]
  LPmethod : Constant  Value=LPmethod
  Math Function1 : Math  Operator=transpose  SaturateOnIntegerOverflow=on
  Math Function2 : Math  Operator=transpose  SaturateOnIntegerOverflow=on
  Math Function3 : Math  Operator=transpose  SaturateOnIntegerOverflow=on
  Matrix Concatenate : Concatenate  Mode=Multidimensional array  ConcatenateDimension=2
  Matrix Concatenate1 : Concatenate  NumInputs=3  Mode=Multidimensional array
  Matrix Concatenate2 : Concatenate  Mode=Multidimensional array  ConcatenateDimension=2
  Matrix Concatenate3 : Concatenate  Mode=Multidimensional array
  Matrix Concatenate4 : Concatenate  Mode=Multidimensional array  ConcatenateDimension=2
  Signal Specification : SignalSpecification  Dimensions=[3 1]
  Signal Specification1 : SignalSpecification  Dimensions=[NumU 1]
  Signal Specification2 : SignalSpecification  Dimensions=[NumU 1]
  Signal Specification3 : SignalSpecification  Dimensions=[NumU 1]
  To Workspace : ToWorkspace  VariableName=INMAT  SampleTime=dt
      settings: MaxDataPoints=1
  Out1 : Outport
  wires:
  Math Function3/1 -> Matrix Concatenate2/1
  Matrix Concatenate2/1 -> Matrix Concatenate1/3
  Signal Specification3/1 -> Math Function3/1
  Bus Selector2/1 -> Signal Specification3/1  "<INDX>"
  LPmethod/1 -> Matrix Concatenate2/2
  Signal Specification2/1 -> Math Function2/1
  Signal Specification1/1 -> Math Function1/1
  Constant2/1 -> Matrix Concatenate4/2
  Matrix Concatenate3/1 -> Matrix Concatenate4/1
  Math Function2/1 -> Matrix Concatenate3/2
  Math Function1/1 -> Matrix Concatenate3/1
  Bus Selector3/2 -> Signal Specification2/1  "<Umax>"
  Bus Selector3/1 -> Signal Specification1/1  "<Umin>"
  Signal Specification/1 -> Matrix Concatenate/2
  Matrix Concatenate4/1 -> Matrix Concatenate1/2
  Matrix Concatenate/1 -> Matrix Concatenate1/1
  Bus Selector1/1 -> Matrix Concatenate/1  "<CB>"
  Bus Selector/1 -> Signal Specification/1  "<CVdt_des>"
  In1/1 -> Bus Selector3/1, Bus Selector2/1, Bus Selector1/1, Bus Selector/1
  Matrix Concatenate1/1 -> Out1/1, To Workspace/1

== system Linear_ADMIRE_sim/ControlAllocation/GetU/MakeSquare_0 ==
  In1 : Inport
  Action Port : ActionPort  ActionType=then
  Bus Selector2 : BusSelector  OutputSignals=CVdt_des
  Divide : Product  Inputs=*/  Multiplication=Matrix(*)
  Product : Product  Multiplication=Matrix(*)
  Subsystem : Subsystem
  Out1 : Outport
  wires:
  Divide/1 -> Product/1
  Bus Selector2/1 -> Product/2  "<CVdt_des>"
  Product/1 -> Out1/1
  In1/1 -> Bus Selector2/1, Subsystem/1(In1)
  Subsystem/1(Gmod) -> Divide/1
  Subsystem/2(CBGmod) -> Divide/2

== system Linear_ADMIRE_sim/ControlAllocation/GetU/VJA_5 ==
  In1 : Inport
  Action Port : ActionPort  ActionType=elseif
  MATLAB Fcn : MATLABFcn  MATLABFcn=VJAwrap(u)
  Out1 : Outport
  wires:
  MATLAB Fcn/1 -> Out1/1
  In1/1 -> MATLAB Fcn/1

== system Linear_ADMIRE_sim/ControlAllocation/GetU/WeightedPseudo Clipped_1 ==
  In1 : Inport
  Action Port : ActionPort  ActionType=elseif
  Bus Selector1 : BusSelector  OutputSignals=CVdt_des
  Constant4 : Constant  Value=Wp
  GetP : Subsystem
  Math Function : Math  Operator=transpose  SaturateOnIntegerOverflow=on
  Math Function1 : Math  Operator=transpose  SaturateOnIntegerOverflow=on
  Product3 : Product  Inputs=**  Multiplication=Matrix(*)  RndMeth=Zero
  SelectActive : Subsystem
  Out1 : Outport
  wires:
  Product3/1 -> Out1/1
  Bus Selector1/1 -> Product3/2  "<CVdt_des>"
  GetP/1(P) -> Product3/1
  Math Function1/1 -> GetP/3(CBT)
  Math Function/1 -> GetP/2(WpT)
  Constant4/1 -> Math Function/1
  In1/1 -> Bus Selector1/1, SelectActive/1(In1)
  SelectActive/1(Out1) -> Math Function1/1, GetP/1(CB)

== system Linear_ADMIRE_sim/ControlAllocation/GetU/WeightedPseudo Scaled_2 ==
  In1 : Inport
  Action Port : ActionPort  ActionType=elseif
  Blocks : Subsystem
  Bus Selector1 : BusSelector  OutputSignals=CVdt_des,Umin,Umax
  Constant4 : Constant  Value=Wp
  Gain : Gain
  SelectActive : Subsystem
  Out1 : Outport
  wires:
  Blocks/1(Out1) -> Gain/1
  Constant4/1 -> Blocks/5(Wp)
  Bus Selector1/3 -> Blocks/4(Umax)  "<Umax>"
  Bus Selector1/2 -> Blocks/3(Umin)  "<Umin>"
  Bus Selector1/1 -> Blocks/2(CVdt_des)  "<CVdt_des>"
  Gain/1 -> Out1/1
  In1/1 -> SelectActive/1(In1), Bus Selector1/1
  SelectActive/1(Out1) -> Blocks/1(CB)

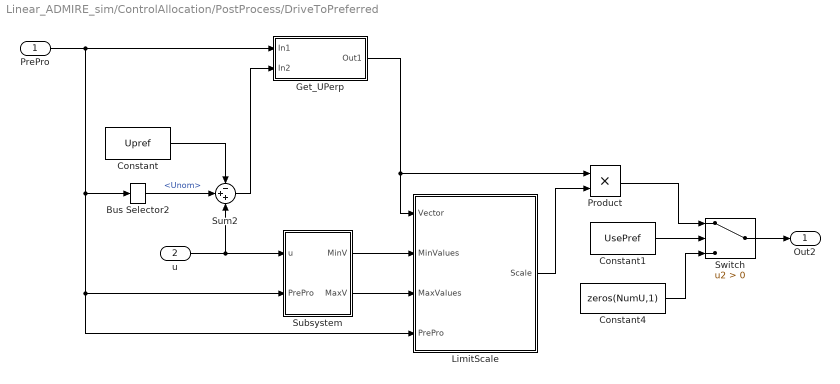
== system Linear_ADMIRE_sim/ControlAllocation/PostProcess/DriveToPreferred ==
  PrePro : Inport
  u : Inport  Port=2
  Bus Selector2 : BusSelector  OutputSignals=Unom
  Constant : Constant  Value=Upref
  Constant1 : Constant  Value=UsePref
  Constant4 : Constant  Value=zeros(NumU,1)
  Get_UPerp : Subsystem
  LimitScale : Subsystem
  Product : Product  RndMeth=Zero
  Subsystem : Subsystem
  Sum2 : Sum  Inputs=-++
  Switch : Switch  Criteria=u2 > Threshold
  Out2 : Outport
  wires:
  u/1 -> Subsystem/1(u), Sum2/3
  PrePro/1 -> Get_UPerp/1(In1), Subsystem/2(PrePro), LimitScale/4(PrePro), Bus Selector2/1
  Bus Selector2/1 -> Sum2/2  "<Unom>"
  LimitScale/1(Scale) -> Product/2
  Subsystem/1(MinV) -> LimitScale/2(MinValues)
  Subsystem/2(MaxV) -> LimitScale/3(MaxValues)
  Constant/1 -> Sum2/1
  Get_UPerp/1(Out1) -> LimitScale/1(Vector), Product/1
  Sum2/1 -> Get_UPerp/2(In2)
  Constant1/1 -> Switch/2
  Switch/1 -> Out2/1
  Product/1 -> Switch/1
  Constant4/1 -> Switch/3

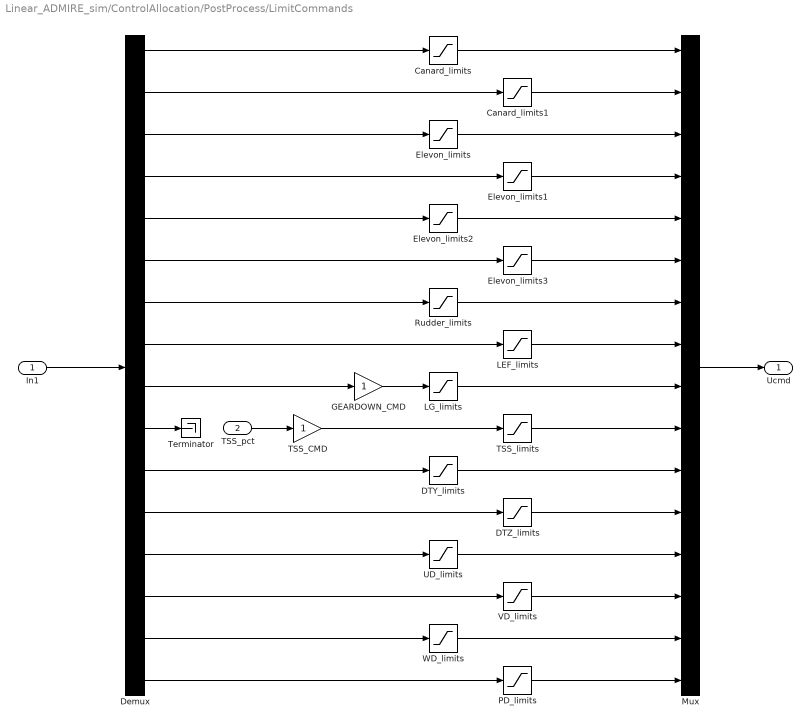
== system Linear_ADMIRE_sim/ControlAllocation/PostProcess/LimitCommands ==
  In1 : Inport
  TSS_pct : Inport  Port=2
  Canard_limits : Saturate  UpperLimit=Canard_max  LowerLimit=Canard_min  RndMeth=Ceiling
  Canard_limits1 : Saturate  UpperLimit=Canard_max  LowerLimit=Canard_min  RndMeth=Ceiling
  DTY_limits : Saturate  UpperLimit=DTY_max  LowerLimit=DTY_min
  DTZ_limits : Saturate  UpperLimit=DTZ_max  LowerLimit=DTZ_min
  Demux : Demux  Outputs=16
  Elevon_limits{,1..3} (4 alike) : Saturate  UpperLimit=Elevon_max  LowerLimit=Elevon_min  RndMeth=Ceiling
  GEARDOWN_CMD : Gain
  LEF_limits : Saturate  UpperLimit=LEF_max  LowerLimit=LEF_min  RndMeth=Ceiling
  LG_limits : Saturate  UpperLimit=LG_max  LowerLimit=LG_min
  Mux : Mux  Inputs=16
  PD_limits : Saturate  UpperLimit=PD_max  LowerLimit=PD_min
  Rudder_limits : Saturate  UpperLimit=Rudder_max  LowerLimit=Rudder_min  RndMeth=Ceiling
  TSS_CMD : Gain
  TSS_limits : Saturate  UpperLimit=TSS_max  LowerLimit=TSS_min
  Terminator : Terminator
  UD_limits : Saturate  UpperLimit=UD_max  LowerLimit=UD_min
  VD_limits : Saturate  UpperLimit=VD_max  LowerLimit=VD_min
  WD_limits : Saturate  UpperLimit=WD_max  LowerLimit=WD_min
  Ucmd : Outport
  wires:
  Demux/7 -> Rudder_limits/1
  Canard_limits1/1 -> Mux/2
  Demux/1 -> Canard_limits/1
  Elevon_limits2/1 -> Mux/5
  Rudder_limits/1 -> Mux/7
  Elevon_limits/1 -> Mux/3
  Elevon_limits1/1 -> Mux/4
  Demux/6 -> Elevon_limits3/1
  Elevon_limits3/1 -> Mux/6
  Mux/1 -> Ucmd/1
  Demux/3 -> Elevon_limits/1
  Demux/2 -> Canard_limits1/1
  Canard_limits/1 -> Mux/1
  Demux/5 -> Elevon_limits2/1
  Demux/4 -> Elevon_limits1/1
  In1/1 -> Demux/1
  DTY_limits/1 -> Mux/11
  DTZ_limits/1 -> Mux/12
  Demux/11 -> DTY_limits/1
  Demux/12 -> DTZ_limits/1
  Demux/13 -> UD_limits/1
  Demux/14 -> VD_limits/1
  Demux/15 -> WD_limits/1
  Demux/16 -> PD_limits/1
  LEF_limits/1 -> Mux/8
  UD_limits/1 -> Mux/13
  VD_limits/1 -> Mux/14
  WD_limits/1 -> Mux/15
  PD_limits/1 -> Mux/16
  Demux/8 -> LEF_limits/1
  Demux/9 -> GEARDOWN_CMD/1
  GEARDOWN_CMD/1 -> LG_limits/1
  TSS_CMD/1 -> TSS_limits/1
  TSS_pct/1 -> TSS_CMD/1
  Demux/10 -> Terminator/1
  TSS_limits/1 -> Mux/10
  LG_limits/1 -> Mux/9

== system Linear_ADMIRE_sim/REGULATORS/PitchReg/CompareTF ==
  Qc : Inport
  Q : Inport  Port=2
  Gain2 : Gain  Gain=r2d
  Gain3 : Gain  Gain=r2d
  Mux1 : Mux  Inputs=2
  QTF_Q : Scope
      settings: TimeRange=10  YMin=-4  YMax=4  SaveName=ScopeData9
  Scope2 : Scope
      settings: TimeRange=10  YMin=-1.5  YMax=1  SaveName=ScopeData10
  Sum2 : Sum  Inputs=|+-
  Transfer Fcn : TransferFcn  Numerator=[(Kfq+Kpq) Kiq]  Denominator=[1 Kpq Kiq]
  Unit Delay : UnitDelay  SampleTime=dt
  wires:
  Transfer Fcn/1 -> Unit Delay/1
  Mux1/1 -> Gain3/1
  Gain3/1 -> QTF_Q/1
  Sum2/1 -> Gain2/1
  Gain2/1 -> Scope2/1
  Qc/1 -> Transfer Fcn/1
  Q/1 -> Mux1/2, Sum2/2
  Unit Delay/1 -> Mux1/1, Sum2/1

== system Linear_ADMIRE_sim/REGULATORS/RollReg/CompareTF ==
  Pc : Inport
  P : Inport  Port=2
  Gain2 : Gain  Gain=r2d
  Gain3 : Gain  Gain=r2d
  Mux1 : Mux  Inputs=2
  PTF_P : Scope
      settings: TimeRange=10  YMin=0  YMax=20  SaveName=ScopeData9
  Scope2 : Scope
      settings: TimeRange=20  YMin=-1  YMax=4  SaveName=ScopeData10
  Sum2 : Sum  Inputs=|+-
  Transfer Fcn : TransferFcn  Numerator=[Kp]  Denominator=[1 Kp]
  Unit Delay : UnitDelay  SampleTime=dt
  wires:
  Transfer Fcn/1 -> Unit Delay/1
  Mux1/1 -> Gain3/1
  Gain3/1 -> PTF_P/1
  Sum2/1 -> Gain2/1
  Gain2/1 -> Scope2/1
  Pc/1 -> Transfer Fcn/1
  P/1 -> Mux1/2, Sum2/2
  Unit Delay/1 -> Mux1/1, Sum2/1

== system Linear_ADMIRE_sim/REGULATORS/YawReg/CompareTF ==
  Rc : Inport
  R : Inport  Port=2
  Gain2 : Gain  Gain=r2d
  Gain3 : Gain  Gain=r2d
  Mux1 : Mux  Inputs=2
  RTF_R : Scope
      settings: TimeRange=10  YMin=0  YMax=150  SaveName=ScopeData9
  Scope2 : Scope
      settings: TimeRange=8  YMin=-0.8  YMax=0.8  SaveName=ScopeData10
  Sum2 : Sum  Inputs=|+-
  Transfer Fcn : TransferFcn  Numerator=[Kr]  Denominator=[1 Kr]
  Unit Delay : UnitDelay  SampleTime=dt
  wires:
  Transfer Fcn/1 -> Unit Delay/1
  Mux1/1 -> Gain3/1
  Gain3/1 -> RTF_R/1
  Sum2/1 -> Gain2/1
  Gain2/1 -> Scope2/1
  Rc/1 -> Transfer Fcn/1
  R/1 -> Mux1/2, Sum2/2
  Unit Delay/1 -> Mux1/1, Sum2/1

== system Linear_ADMIRE_sim/ControlAllocation/GetU/MakeSquare_0/Subsystem ==
  In1 : Inport
  Bus Selector1 : BusSelector  OutputSignals=CB
  Bus Selector3 : BusSelector  OutputSignals=INDX
  Constant : Constant  Value=G
  Math Function2 : Math  Operator=transpose  SaturateOnIntegerOverflow=on
  Matrix Concatenate : Concatenate  NumInputs=3  Mode=Multidimensional array
  Product : Product
  Product1 : Product  Multiplication=Matrix(*)
  Signal Specification1 : SignalSpecification  Dimensions=[1 NumU]
  Gmod : Outport
  CBGmod : Outport  Port=2
  wires:
  Math Function2/1 -> Product/2
  Bus Selector3/1 -> Signal Specification1/1  "<INDX>"
  Signal Specification1/1 -> Matrix Concatenate/1, Matrix Concatenate/2, Matrix Concatenate/3
  Product/1 -> Product1/2, Gmod/1
  Matrix Concatenate/1 -> Math Function2/1
  Constant/1 -> Product/1
  Bus Selector1/1 -> Product1/1  "<CB>"
  In1/1 -> Bus Selector1/1, Bus Selector3/1
  Product1/1 -> CBGmod/1

== system Linear_ADMIRE_sim/ControlAllocation/GetU/WeightedPseudo Clipped_1/GetP ==
  CB : Inport
  WpT : Inport  Port=2
  CBT : Inport  Port=3
  Product : Product  Inputs=/*  Multiplication=Matrix(*)  RndMeth=Zero
  Product1 : Product  Inputs=**  Multiplication=Matrix(*)  RndMeth=Zero
  Product2 : Product  Inputs=*/  Multiplication=Matrix(*)  RndMeth=Zero
  P : Outport
  wires:
  CBT/1 -> Product/2
  Product2/1 -> P/1  "P"
  WpT/1 -> Product/1
  CB/1 -> Product1/1
  Product1/1 -> Product2/2
  Product/1 -> Product2/1, Product1/2

== system Linear_ADMIRE_sim/ControlAllocation/GetU/WeightedPseudo Clipped_1/SelectActive ==
  In1 : Inport
  Bus Selector2 : BusSelector  OutputSignals=CB
  Bus Selector3 : BusSelector  OutputSignals=INDX
  Matrix Concatenate : Concatenate  NumInputs=3  Mode=Multidimensional array
  Product : Product
  Signal Specification1 : SignalSpecification  Dimensions=[1 NumU]
  Out1 : Outport
  wires:
  Matrix Concatenate/1 -> Product/1
  Product/1 -> Out1/1
  Bus Selector3/1 -> Signal Specification1/1  "<INDX>"
  Bus Selector2/1 -> Product/2  "<CB>"
  In1/1 -> Bus Selector3/1, Bus Selector2/1
  Signal Specification1/1 -> Matrix Concatenate/3, Matrix Concatenate/2, Matrix Concatenate/1

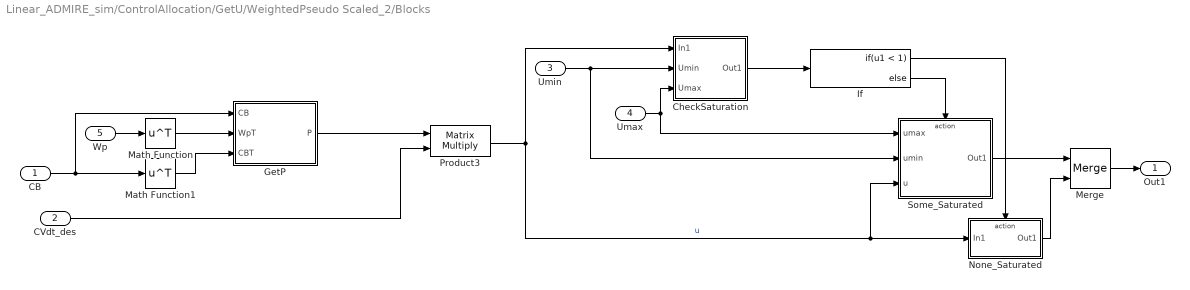
== system Linear_ADMIRE_sim/ControlAllocation/GetU/WeightedPseudo Scaled_2/Blocks ==
  CB : Inport
  CVdt_des : Inport  Port=2
  Umin : Inport  Port=3
  Umax : Inport  Port=4
  Wp : Inport  Port=5
  CheckSaturation : Subsystem
  GetP : Subsystem
  If : If  IfExpression=u1 < 1
  Math Function : Math  Operator=transpose  SaturateOnIntegerOverflow=on
  Math Function1 : Math  Operator=transpose  SaturateOnIntegerOverflow=on
  Merge : Merge
  None_Saturated : Subsystem  TreatAsAtomicUnit=on
  Product3 : Product  Inputs=**  Multiplication=Matrix(*)  RndMeth=Zero
  Some_Saturated : Subsystem  TreatAsAtomicUnit=on
  Out1 : Outport
  wires:
  Merge/1 -> Out1/1
  Umin/1 -> Some_Saturated/2(umin), CheckSaturation/2(Umin)
  Umax/1 -> Some_Saturated/1(umax), CheckSaturation/3(Umax)
  None_Saturated/1(Out1) -> Merge/2
  Some_Saturated/1(Out1) -> Merge/1
  If/1 -> None_Saturated/Action
  If/2 -> Some_Saturated/Action
  CheckSaturation/1(Out1) -> If/1
  Product3/1 -> CheckSaturation/1(In1), Some_Saturated/3(u), None_Saturated/1(In1)  "u"
  CVdt_des/1 -> Product3/2
  GetP/1(P) -> Product3/1
  Math Function1/1 -> GetP/3(CBT)
  Math Function/1 -> GetP/2(WpT)
  Wp/1 -> Math Function/1
  CB/1 -> GetP/1(CB), Math Function1/1

== system Linear_ADMIRE_sim/ControlAllocation/GetU/WeightedPseudo Scaled_2/SelectActive ==
  In1 : Inport
  Bus Selector2 : BusSelector  OutputSignals=CB
  Bus Selector3 : BusSelector  OutputSignals=INDX
  Matrix Concatenate : Concatenate  NumInputs=3  Mode=Multidimensional array
  Product : Product
  Signal Specification1 : SignalSpecification  Dimensions=[1 NumU]
  Out1 : Outport
  wires:
  Matrix Concatenate/1 -> Product/1
  Product/1 -> Out1/1
  Bus Selector3/1 -> Signal Specification1/1  "<INDX>"
  Bus Selector2/1 -> Product/2  "<CB>"
  In1/1 -> Bus Selector3/1, Bus Selector2/1
  Signal Specification1/1 -> Matrix Concatenate/3, Matrix Concatenate/2, Matrix Concatenate/1

== system Linear_ADMIRE_sim/ControlAllocation/PostProcess/DriveToPreferred/Get_UPerp ==
  In1 : Inport
  In2 : Inport  Port=2
  Bus Selector3 : BusSelector  OutputSignals=CB,INDX
  MATLAB Fcn : MATLABFcn  MATLABFcn=getUperp  Output1D=off
  Math Function1 : Math  Operator=transpose  SaturateOnIntegerOverflow=on
  Math Function3 : Math  Operator=transpose  SaturateOnIntegerOverflow=on
  Matrix Concatenate : Concatenate  NumInputs=3  Mode=Multidimensional array
  Signal Specification1 : SignalSpecification  Dimensions=[NumU 1]
  Signal Specification3 : SignalSpecification  Dimensions=[NumU 1]
  Out1 : Outport
  wires:
  Signal Specification3/1 -> Math Function3/1
  Matrix Concatenate/1 -> MATLAB Fcn/1
  In1/1 -> Bus Selector3/1
  Bus Selector3/2 -> Signal Specification3/1  "<INDX>"
  MATLAB Fcn/1 -> Out1/1
  Bus Selector3/1 -> Matrix Concatenate/1  "<CB>"
  In2/1 -> Signal Specification1/1
  Signal Specification1/1 -> Math Function1/1
  Math Function1/1 -> Matrix Concatenate/2
  Math Function3/1 -> Matrix Concatenate/3

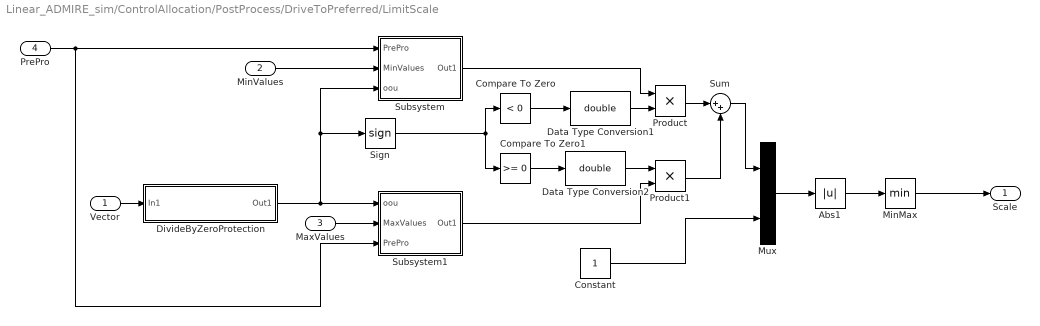
== system Linear_ADMIRE_sim/ControlAllocation/PostProcess/DriveToPreferred/LimitScale ==
  Vector : Inport
  MinValues : Inport  Port=2
  MaxValues : Inport  Port=3
  PrePro : Inport  Port=4
  Abs1 : Abs
  Compare To Zero : simulink/Logic and Bit Operations/Compare To Zero  relop=<  OutDataTypeStr=uint8
  Compare To Zero1 : simulink/Logic and Bit Operations/Compare To Zero  relop=>=  OutDataTypeStr=uint8
  Constant : Constant
  Data Type Conversion1 : DataTypeConversion  OutDataTypeStr=double
  Data Type Conversion2 : DataTypeConversion  OutDataTypeStr=double
  DivideByZeroProtection : Subsystem
  MinMax : MinMax
  Mux : Mux  Inputs=2
  Product : Product  RndMeth=Zero
  Product1 : Product  RndMeth=Zero
  Sign : Signum
  Subsystem : Subsystem
  Subsystem1 : Subsystem
  Sum : Sum  Inputs=|++
  Scale : Outport
  wires:
  Abs1/1 -> MinMax/1
  MinMax/1 -> Scale/1
  Vector/1 -> DivideByZeroProtection/1(In1)
  DivideByZeroProtection/1(Out1) -> Subsystem1/1(oou), Sign/1, Subsystem/3(oou)
  MaxValues/1 -> Subsystem1/2(MaxValues)
  Mux/1 -> Abs1/1
  Constant/1 -> Mux/2
  PrePro/1 -> Subsystem1/3(PrePro), Subsystem/1(PrePro)
  MinValues/1 -> Subsystem/2(MinValues)
  Sign/1 -> Compare To Zero/1, Compare To Zero1/1
  Compare To Zero/1 -> Data Type Conversion1/1
  Data Type Conversion1/1 -> Product/2
  Subsystem/1(Out1) -> Product/1
  Product/1 -> Sum/1
  Compare To Zero1/1 -> Data Type Conversion2/1
  Data Type Conversion2/1 -> Product1/1
  Subsystem1/1(Out1) -> Product1/2
  Product1/1 -> Sum/2
  Sum/1 -> Mux/1

== system Linear_ADMIRE_sim/ControlAllocation/PostProcess/DriveToPreferred/Subsystem ==
  u : Inport
  PrePro : Inport  Port=2
  Bus Selector1 : BusSelector  OutputSignals=Umax
  Bus Selector3 : BusSelector  OutputSignals=Umin
  Sum1 : Sum  Inputs=-+|
  Sum4 : Sum  Inputs=|+-
  MinV : Outport
  MaxV : Outport  Port=2
  wires:
  Bus Selector3/1 -> Sum4/1  "<Umin>"
  PrePro/1 -> Bus Selector3/1, Bus Selector1/1
  Sum4/1 -> MinV/1
  u/1 -> Sum4/2, Sum1/1
  Bus Selector1/1 -> Sum1/2  "<Umax>"
  Sum1/1 -> MaxV/1

== system Linear_ADMIRE_sim/ControlAllocation/GetU/WeightedPseudo Scaled_2/Blocks/CheckSaturation ==
  In1 : Inport
  Umin : Inport  Port=2
  Umax : Inport  Port=3
  Relational Operator : RelationalOperator  Operator=<  OutDataTypeStr=boolean
  Relational Operator1 : RelationalOperator  Operator=>  OutDataTypeStr=boolean
  Sum : Sum  Inputs=|++
  Sum of Elements : Sum  Inputs=+
  Sum of Elements1 : Sum  Inputs=+
  Out1 : Outport
  wires:
  Sum/1 -> Out1/1
  In1/1 -> Relational Operator/1, Relational Operator1/1
  Sum of Elements1/1 -> Sum/2
  Sum of Elements/1 -> Sum/1
  Relational Operator/1 -> Sum of Elements1/1
  Relational Operator1/1 -> Sum of Elements/1
  Umax/1 -> Relational Operator1/2
  Umin/1 -> Relational Operator/2

== system Linear_ADMIRE_sim/ControlAllocation/GetU/WeightedPseudo Scaled_2/Blocks/GetP ==
  CB : Inport
  WpT : Inport  Port=2
  CBT : Inport  Port=3
  Product : Product  Inputs=/*  Multiplication=Matrix(*)  RndMeth=Zero
  Product1 : Product  Inputs=**  Multiplication=Matrix(*)  RndMeth=Zero
  Product2 : Product  Inputs=*/  Multiplication=Matrix(*)  RndMeth=Zero
  P : Outport
  wires:
  CBT/1 -> Product/2
  Product2/1 -> P/1  "P"
  WpT/1 -> Product/1
  CB/1 -> Product1/1
  Product1/1 -> Product2/2
  Product/1 -> Product2/1, Product1/2

== system Linear_ADMIRE_sim/ControlAllocation/GetU/WeightedPseudo Scaled_2/Blocks/None_Saturated ==
  In1 : Inport
  Action Port : ActionPort  ActionType=then
  Out1 : Outport
  wires:
  In1/1 -> Out1/1

== system Linear_ADMIRE_sim/ControlAllocation/GetU/WeightedPseudo Scaled_2/Blocks/Some_Saturated ==
  umax : Inport
  umin : Inport  Port=2
  u : Inport  Port=3
  Action Port : ActionPort  ActionType=else
  For Iterator Subsystem : Subsystem  TreatAsAtomicUnit=on
  Product : Product  RndMeth=Zero
  Out1 : Outport
  wires:
  Product/1 -> Out1/1
  For Iterator Subsystem/1(Out1) -> Product/2
  umin/1 -> For Iterator Subsystem/3(umin)
  umax/1 -> For Iterator Subsystem/2(umax)
  u/1 -> Product/1, For Iterator Subsystem/1(u)

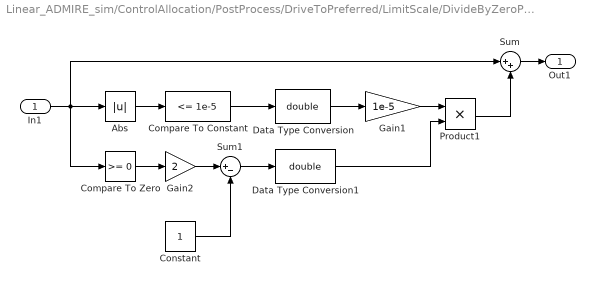
== system Linear_ADMIRE_sim/ControlAllocation/PostProcess/DriveToPreferred/LimitScale/DivideByZeroProtection ==
  In1 : Inport
  Abs : Abs
  Compare To Constant : simulink/Logic and Bit Operations/Compare To Constant  relop=<=  const=1e-5  OutDataTypeStr=uint8
  Compare To Zero : simulink/Logic and Bit Operations/Compare To Zero  relop=>=  OutDataTypeStr=uint8
  Constant : Constant
  Data Type Conversion : DataTypeConversion  OutDataTypeStr=double
  Data Type Conversion1 : DataTypeConversion  OutDataTypeStr=double
  Gain1 : Gain  Gain=1e-5
  Gain2 : Gain  Gain=2
  Product1 : Product  RndMeth=Zero
  Sum : Sum  Inputs=|++
  Sum1 : Sum  Inputs=|+-
  Out1 : Outport
  wires:
  Abs/1 -> Compare To Constant/1
  Data Type Conversion/1 -> Gain1/1
  Gain1/1 -> Product1/1
  Sum1/1 -> Data Type Conversion1/1
  Compare To Zero/1 -> Gain2/1
  Gain2/1 -> Sum1/1
  Constant/1 -> Sum1/2
  Data Type Conversion1/1 -> Product1/2
  Compare To Constant/1 -> Data Type Conversion/1
  In1/1 -> Sum/1, Compare To Zero/1, Abs/1
  Product1/1 -> Sum/2
  Sum/1 -> Out1/1

== system Linear_ADMIRE_sim/ControlAllocation/PostProcess/DriveToPreferred/LimitScale/Subsystem ==
  PrePro : Inport
  MinValues : Inport  Port=2
  oou : Inport  Port=3
  Bus Selector2 : BusSelector  OutputSignals=INDX
  Compare To Constant : simulink/Logic and Bit Operations/Compare To Constant  relop=<=  const=0.5  OutDataTypeStr=uint8
  Data Type Conversion : DataTypeConversion  OutDataTypeStr=double
  Product : Product  Inputs=*/  RndMeth=Zero
  Product2 : Product
  Sum : Sum  Inputs=|++
  Out1 : Outport
  wires:
  Product/1 -> Product2/2
  oou/1 -> Product/2
  Sum/1 -> Out1/1
  MinValues/1 -> Product/1
  PrePro/1 -> Bus Selector2/1
  Product2/1 -> Sum/2
  Bus Selector2/1 -> Compare To Constant/1, Product2/1  "<INDX>"
  Data Type Conversion/1 -> Sum/1
  Compare To Constant/1 -> Data Type Conversion/1

== system Linear_ADMIRE_sim/ControlAllocation/PostProcess/DriveToPreferred/LimitScale/Subsystem1 ==
  oou : Inport
  MaxValues : Inport  Port=2
  PrePro : Inport  Port=3
  Bus Selector2 : BusSelector  OutputSignals=INDX
  Compare To Constant : simulink/Logic and Bit Operations/Compare To Constant  relop=<=  const=0.5  OutDataTypeStr=uint8
  Data Type Conversion : DataTypeConversion  OutDataTypeStr=double
  Product : Product  Inputs=*/  RndMeth=Zero
  Product2 : Product
  Sum : Sum  Inputs=|++
  Out1 : Outport
  wires:
  Compare To Constant/1 -> Data Type Conversion/1
  Data Type Conversion/1 -> Sum/1
  Bus Selector2/1 -> Product2/1, Compare To Constant/1  "<INDX>"
  Product2/1 -> Sum/2
  PrePro/1 -> Bus Selector2/1
  MaxValues/1 -> Product/1
  Sum/1 -> Out1/1
  oou/1 -> Product/2
  Product/1 -> Product2/2

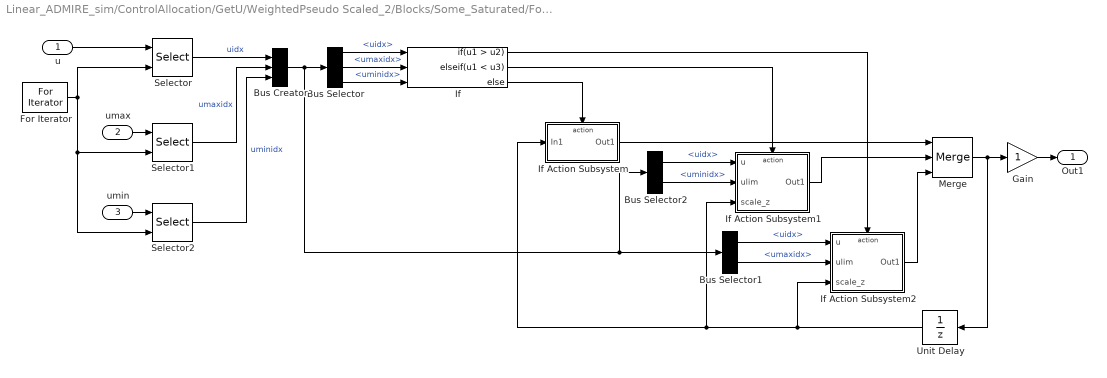
== system Linear_ADMIRE_sim/ControlAllocation/GetU/WeightedPseudo Scaled_2/Blocks/Some_Saturated/For Iterator Subsystem ==
  u : Inport
  umax : Inport  Port=2
  umin : Inport  Port=3
  Bus Creator : BusCreator  Inputs=3
  Bus Selector : BusSelector  OutputSignals=uidx,umaxidx,uminidx
  Bus Selector1 : BusSelector  OutputSignals=uidx,umaxidx
  Bus Selector2 : BusSelector  OutputSignals=uidx,uminidx
  For Iterator : ForIterator  IterationLimit=7
  Gain : Gain
  If : If  NumInputs=3  IfExpression=u1 > u2  ElseIfExpressions=u1 < u3
  If Action Subsystem : Subsystem  TreatAsAtomicUnit=on
  If Action Subsystem1 : Subsystem  TreatAsAtomicUnit=on
  If Action Subsystem2 : Subsystem  TreatAsAtomicUnit=on
  Merge : Merge  Inputs=3
  Selector : Selector  IndexOptions=Index vector (port)  Indices=[1 3]
  Selector1 : Selector  IndexOptions=Index vector (port)  Indices=[1 3]
  Selector2 : Selector  IndexOptions=Index vector (port)  Indices=[1 3]
  Unit Delay : UnitDelay  InitialCondition=1  SampleTime=-1
  Out1 : Outport
  wires:
  Bus Selector2/2 -> If Action Subsystem1/2(ulim)  "<uminidx>"
  Bus Selector2/1 -> If Action Subsystem1/1(u)  "<uidx>"
  Bus Selector1/2 -> If Action Subsystem2/2(ulim)  "<umaxidx>"
  Bus Selector1/1 -> If Action Subsystem2/1(u)  "<uidx>"
  Bus Selector/3 -> If/3  "<uminidx>"
  Bus Selector/2 -> If/2  "<umaxidx>"
  Bus Selector/1 -> If/1  "<uidx>"
  Bus Creator/1 -> Bus Selector/1, Bus Selector2/1, Bus Selector1/1
  Unit Delay/1 -> If Action Subsystem2/3(scale_z), If Action Subsystem/1(In1), If Action Subsystem1/3(scale_z)
  Merge/1 -> Unit Delay/1, Gain/1
  If Action Subsystem1/1(Out1) -> Merge/2
  If Action Subsystem2/1(Out1) -> Merge/3
  If Action Subsystem/1(Out1) -> Merge/1
  If/1 -> If Action Subsystem2/Action
  If/2 -> If Action Subsystem1/Action
  If/3 -> If Action Subsystem/Action
  Selector2/1 -> Bus Creator/3  "uminidx"
  Selector1/1 -> Bus Creator/2  "umaxidx"
  Selector/1 -> Bus Creator/1  "uidx"
  umin/1 -> Selector2/1
  umax/1 -> Selector1/1
  Gain/1 -> Out1/1
  For Iterator/1 -> Selector2/2, Selector1/2, Selector/2
  u/1 -> Selector/1

== system Linear_ADMIRE_sim/ControlAllocation/GetU/WeightedPseudo Scaled_2/Blocks/Some_Saturated/For Iterator Subsystem/If Action Subsystem ==
  In1 : Inport
  Action Port : ActionPort  ActionType=else
  Out1 : Outport
  wires:
  In1/1 -> Out1/1

== system Linear_ADMIRE_sim/ControlAllocation/GetU/WeightedPseudo Scaled_2/Blocks/Some_Saturated/For Iterator Subsystem/If Action Subsystem1 ==
  u : Inport
  ulim : Inport  Port=2
  scale_z : Inport  Port=3
  Action Port : ActionPort  ActionType=elseif
  Abs : Abs
  If : If  IfExpression=u1 >1e-5
  If Action Subsystem : Subsystem  TreatAsAtomicUnit=on
  If Action Subsystem1 : Subsystem  TreatAsAtomicUnit=on
  Merge : Merge
  Out1 : Outport
  wires:
  If Action Subsystem/1(Out1) -> Merge/2
  If/1 -> If Action Subsystem/Action
  If Action Subsystem1/1(Out1) -> Merge/1
  If/2 -> If Action Subsystem1/Action
  scale_z/1 -> If Action Subsystem/3(scale_z)
  ulim/1 -> If Action Subsystem/2(ulim)
  Merge/1 -> Out1/1
  u/1 -> If Action Subsystem/1(u), Abs/1
  Abs/1 -> If/1

== system Linear_ADMIRE_sim/ControlAllocation/GetU/WeightedPseudo Scaled_2/Blocks/Some_Saturated/For Iterator Subsystem/If Action Subsystem2 ==
  u : Inport
  ulim : Inport  Port=2
  scale_z : Inport  Port=3
  Action Port : ActionPort  ActionType=then
  Abs : Abs
  If : If  IfExpression=u1 >1e-5
  If Action Subsystem : Subsystem  TreatAsAtomicUnit=on
  If Action Subsystem1 : Subsystem  TreatAsAtomicUnit=on
  Merge : Merge
  Out1 : Outport
  wires:
  If Action Subsystem/1(Out1) -> Merge/2
  If/1 -> If Action Subsystem/Action
  If Action Subsystem1/1(Out1) -> Merge/1
  If/2 -> If Action Subsystem1/Action
  scale_z/1 -> If Action Subsystem/3(scale_z)
  ulim/1 -> If Action Subsystem/2(ulim)
  Merge/1 -> Out1/1
  u/1 -> If Action Subsystem/1(u), Abs/1
  Abs/1 -> If/1
